simulink model "LV_grid"  (R2021b)
settings: Solver=VariableStepAuto  StartTime=0  StopTime=5.0005  FixedStep=5e-4  RelTol=1e-3
model workspace (MAT data in the model file):
  P2_1 = 3450
  idx = 1
  time_counter = 1
libraries: spsGroundLib x97, spsStairGeneratorLib x96, spsPiSectionLineLib x90, spsThreePhasePISectionLineLib x90, spsVariableInductorLib x48, spsVariableResistorLib x48, spsRMSLib x36, spsThreePhaseVIMeasurementLib x34, spsACVoltageSourceLib x5, spsLinearTransformerLib x5, spsPower3phInstantaneousLib x1, spsThreePhaseMutualInductanceZ1Z0Lib x1
(part 1 of 6)
settings Model: Creator=vasri  LastModifiedBy=vasri
settings SolverCC: AlgebraicLoopSolver=TrustRegion
settings DataIOCC: FinalStateName=LV_grid_ctx01  SaveFinalState=on  SaveOperatingPoint=on
settings DebuggingCC: SFMachineParentedDataDiag=warning

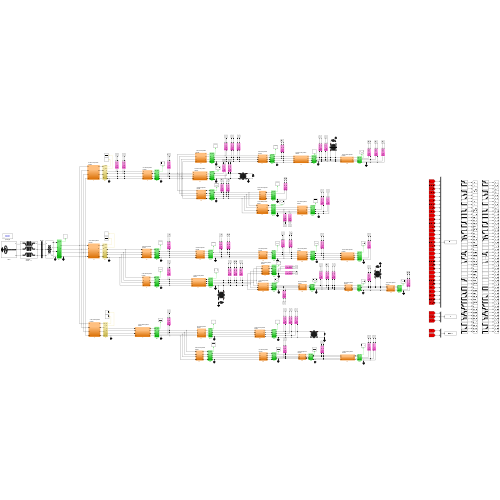
[thumbnail: Simulink's stored preview of the top-level diagram]
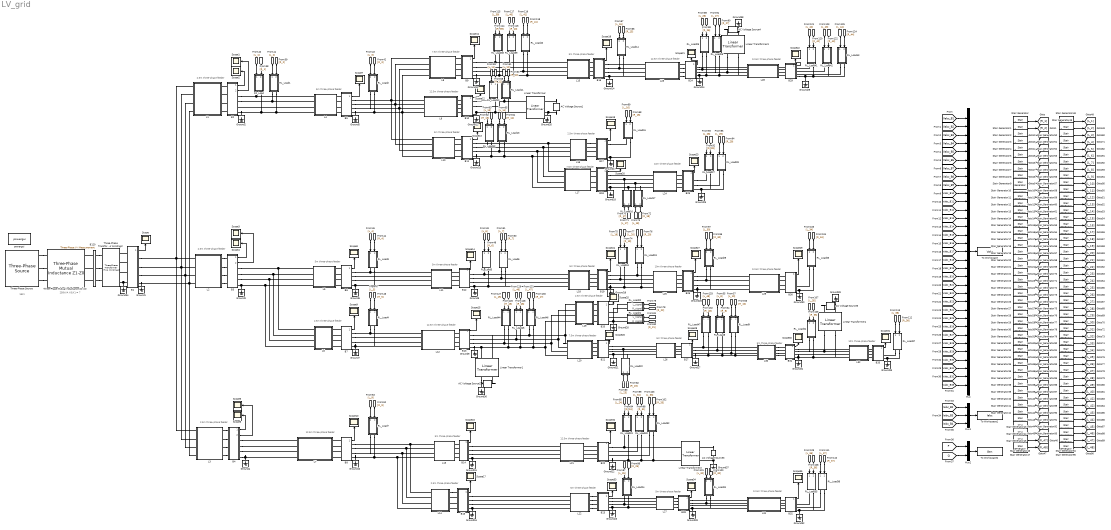
== system LV_grid ==
  note: 12.5m three-phase
      | feeder
  note: 2.5m three-phase
      | feeder
  note: 5m three-phase
      | feeder
  note: 15kV
  note: 250kVA
      | Χ0/Χ1 = 7
  note: 7.5m three-phase
      | feeder
  note: 10m three-phase
      | feeder
  note: 2.5m three-phase
      | feeder
  note: 2.5m three-phase
      | feeder
  note: 2.5m three-phase
      | feeder
  note: 2.5m three-phase
      | feeder
  note: 5m three-phase
      | feeder
  note: 5m three-phase
      | feeder
  note: 5m three-phase
      | feeder
  note: 5m three-phase
      | feeder
  note: 5m three-phase
      | feeder
  note: 5m three-phase
      | feeder
  note: 5m three-phase
      | feeder
  note: 5m three-phase
      | feeder
  note: 5m three-phase
      | feeder
  note: 5m three-phase
      | feeder
  note: 7.5m three-phase
      | feeder
  note: 7.5m three-phase
      | feeder
  note: 10m three-phase
      | feeder
  note: 10m three-phase
      | feeder
  note: 12.5m three-phase
      | feeder
  note: 12.5m three-phase
      | feeder
  note: 12.5m three-phase
      | feeder
  note: 12.5m three-phase
      | feeder
  note: 12.5m three-phase
      | feeder
  note: 12.5m three-phase
      | feeder
  note: 12.5m three-phase
      | feeder
  note: 2.5m three-phase
      | feeder
  note: 2.5m three-phase
      | feeder
  " B120" : spsThreePhaseVIMeasurementLib/Three-Phase V-I Measurement  VoltageMeasurement=no  SetLabelV=off  LabelV=Vabc  Vpu=off  VpuLL=off  CurrentMeasurement=no  SetLabelI=off  LabelI=Iabc  Ipu=on  Pbase=100e6  Vbase=1  OutputType=Complex  PhasorSimulation=off  PSBequivalent=0
  AC Voltage Source1 : spsACVoltageSourceLib/AC Voltage Source  Amplitude=325.27  Phase=-120  Frequency=50  SampleTime=0  Measurements=None  BusType=PV  Pref=6596.9588  Qref=0  Qmin=-inf  Qmax=+inf
  AC Voltage Source2 : spsACVoltageSourceLib/AC Voltage Source  Amplitude=325.27  Phase=0  Frequency=50  SampleTime=0  Measurements=None  BusType=PV  Pref=4239.5175  Qref=0  Qmin=-inf  Qmax=+inf
  AC Voltage Source3 : spsACVoltageSourceLib/AC Voltage Source  Amplitude=325.27  Phase=0  Frequency=50  SampleTime=0  Measurements=None  BusType=PV  Pref=2354.85  Qref=0  Qmin=-inf  Qmax=+inf
  AC Voltage Source4 : spsACVoltageSourceLib/AC Voltage Source  Amplitude=325.27  Phase=120  Frequency=50  SampleTime=0  Measurements=None  BusType=PV  Pref=9631.012  Qref=0  Qmin=-inf  Qmax=+inf
  AC Voltage Source5 : spsACVoltageSourceLib/AC Voltage Source  Amplitude=325.27  Phase=-120  Frequency=50  SampleTime=0  Measurements=None  BusType=PV  Pref=3979.8713  Qref=0  Qmin=-inf  Qmax=+inf
  B1 : Subsystem
  B10 : Subsystem
  B11 : Subsystem
  B12 : Subsystem
  B13 : Subsystem
  B14 : Subsystem
  B15 : Subsystem
  B16 : Subsystem
  B17 : Subsystem
  B18 : Subsystem
  B19 : Subsystem
  B2 : Subsystem
  B20 : Subsystem
  B21 : Subsystem
  B22 : Subsystem
  B23 : Subsystem
  B24 : Subsystem
  B25 : Subsystem
  B26 : Subsystem
  B27 : Subsystem
  B28 : Subsystem
  B29 : Subsystem
  B3 : Subsystem
  B30 : Subsystem
  B31 : Subsystem
  B32 : Subsystem
  B33 : Subsystem
  B4 : Subsystem
  B5 : Subsystem
  B6 : Subsystem
  B7 : Subsystem
  B8 : Subsystem
  B9 : Subsystem
  Ground{1..39} (39 alike) : spsGroundLib/Ground  LConnTagsString=a
  L1 : Subsystem
  L10 : Subsystem
  L11 : Subsystem
  L12 : Subsystem
  L13 : Subsystem
  L14 : Subsystem
  L15 : Subsystem
  L16 : Subsystem
  L17 : Subsystem
  L18 : Subsystem
  L19 : Subsystem
  L2 : Subsystem
  L20 : Subsystem
  L21 : Subsystem
  L22 : Subsystem
  L23 : Subsystem
  L24 : Subsystem
  L25 : Subsystem
  L26 : Subsystem
  L27 : Subsystem
  L28 : Subsystem
  L29 : Subsystem
  L3 : Subsystem
  L30 : Subsystem
  L31 : Subsystem
  L32 : Subsystem
  L4 : Subsystem
  L5 : Subsystem
  L6 : Subsystem
  L7 : Subsystem
  L8 : Subsystem
  L9 : Subsystem
  Linear Transformer{,1..4} (5 alike) : spsLinearTransformerLib/Linear Transformer  UNITS=pu  NominalPower=[ 3680 50 ]  winding1="[ 400  0.002  0.08 ]"  winding2="[ 400  0.002  0.08 ]"  ThreeWindings=off  winding3=[ 315e3 0.002 0.08 ]  RmLm=[ 500 500 ]  Measurements=None  DataType=off
  Mux : Mux  Inputs=33
  Mux1 : Mux  Inputs=3
  Mux2 : Mux  Inputs=2
  RL_Load : Subsystem
  RL_Load1 : Subsystem
  RL_Load10 : Subsystem
  RL_Load11 : Subsystem
  RL_Load12 : Subsystem
  RL_Load13 : Subsystem
  RL_Load14 : Subsystem
  RL_Load15 : Subsystem
  RL_Load16 : Subsystem
  RL_Load17 : Subsystem
  RL_Load18 : Subsystem
  RL_Load19 : Subsystem
  RL_Load2 : Subsystem
  RL_Load20 : Subsystem
  RL_Load21 : Subsystem
  RL_Load22 : Subsystem
  RL_Load23 : Subsystem
  RL_Load24 : Subsystem
  RL_Load25 : Subsystem
  RL_Load26 : Subsystem
  RL_Load27 : Subsystem
  RL_Load28 : Subsystem
  RL_Load29 : Subsystem
  RL_Load3 : Subsystem
  RL_Load30 : Subsystem
  RL_Load31 : Subsystem
  RL_Load32 : Subsystem
  RL_Load33 : Subsystem
  RL_Load34 : Subsystem
  RL_Load35 : Subsystem
  RL_Load36 : Subsystem
  RL_Load37 : Subsystem
  RL_Load38 : Subsystem
  RL_Load39 : Subsystem
  RL_Load4 : Subsystem
  RL_Load40 : Subsystem
  RL_Load41 : Subsystem
  RL_Load42 : Subsystem
  RL_Load43 : Subsystem
  RL_Load44 : Subsystem
  RL_Load45 : Subsystem
  RL_Load46 : Subsystem
  RL_Load47 : Subsystem
  RL_Load5 : Subsystem
  RL_Load6 : Subsystem
  RL_Load7 : Subsystem
  RL_Load8 : Subsystem
  RL_Load9 : Subsystem
  Scope{,1..35} (36 alike) : Scope
  Stair Generator : spsStairGeneratorLib/Stair Generator  t=[0,2.617,3.6925,4.8825]  e=[168.7617,168.5927,168.424,168.2557]  Ts=0.0005
  Stair Generator1 : spsStairGeneratorLib/Stair Generator  t=[0,1.0365,2.15]  e=[73.2041,70.2093,67.4499]  Ts=0.0005
  Stair Generator10 : spsStairGeneratorLib/Stair Generator  t=[0,1.492,2.483]  e=[35.5387,35.625,35.7117]  Ts=0.0005
  Stair Generator11 : spsStairGeneratorLib/Stair Generator  t=[0,2.5075,4.45]  e=[24.3172,26.1566,28.2971]  Ts=0.0005
  Stair Generator12 : spsStairGeneratorLib/Stair Generator  t=[0,1.3855]  e=[0,0]  Ts=0.0005
  Stair Generator13 : spsStairGeneratorLib/Stair Generator  t=[0,0.0745,2.0645,2.6705,2.8715]  e=[353.8462,353.7729,353.6997,353.6265,353.5533]  Ts=0.0005
  Stair Generator14 : spsStairGeneratorLib/Stair Generator  t=[0,2.534,3.5145]  e=[220.7485,220.5687,220.3893]  Ts=0.0005
  Stair Generator15 : spsStairGeneratorLib/Stair Generator  t=[0,0.325,1.7935,1.907]  e=[979.2809,980.7642,982.2521,983.7445]  Ts=0.0005
  Stair Generator16 : spsStairGeneratorLib/Stair Generator  t=[0,1.018,1.172,1.9675,4.0695]  e=[234.6084,234.5768,234.5452,234.5136,234.4821]  Ts=0.0005
  Stair Generator17 : spsStairGeneratorLib/Stair Generator  t=[0,0.2685,1.876,3.8755]  e=[98.0581,98.0807,98.1032,98.1258]  Ts=0.0005
  Stair Generator18 : spsStairGeneratorLib/Stair Generator  t=[0,0.827,1.5965,4.5615]  e=[253.6736,253.7195,253.7655,253.8114]  Ts=0.0005
  Stair Generator19 : spsStairGeneratorLib/Stair Generator  t=[0,1.6495]  e=[0,0]  Ts=0.0005
  Stair Generator2 : spsStairGeneratorLib/Stair Generator  t=[0,1.6175]  e=[0,0]  Ts=0.0005
  Stair Generator20 : spsStairGeneratorLib/Stair Generator  t=[0,0.3505,1.0215,3.8365]  e=[6.1612,6.1612,6.1612,6.1612]  Ts=0.0005
  Stair Generator21 : spsStairGeneratorLib/Stair Generator  t=[0,0.7915,1.4325,3.436,4.7505]  e=[113.7634,113.7634,113.7634,113.7634,113.7634]  Ts=0.0005
  Stair Generator22 : spsStairGeneratorLib/Stair Generator  t=[0,0.706,2.561,3.607]  e=[126.7148,126.7293,126.7438,126.7584]  Ts=0.0005
  Stair Generator23 : spsStairGeneratorLib/Stair Generator  t=[0,2.037,3.661,3.7495,4.6445]  e=[58.0436,58.0068,57.9701,57.9334,57.8968]  Ts=0.0005
  Stair Generator24 : spsStairGeneratorLib/Stair Generator  t=[0,1.096,1.198,2.605,4.2125]  e=[288.4476,288.4443,288.4409,288.4376,288.4343]  Ts=0.0005
  Stair Generator25 : spsStairGeneratorLib/Stair Generator  t=[0,2.346,3.315,3.97,4.0815]  e=[48.1074,48.1096,48.1118,48.114,48.1162]  Ts=0.0005
  Stair Generator26 : spsStairGeneratorLib/Stair Generator  t=[0,1.548]  e=[0,0]  Ts=0.0005
  Stair Generator27 : spsStairGeneratorLib/Stair Generator  t=[0,3.4385]  e=[0,0]  Ts=0.0005
  Stair Generator28 : spsStairGeneratorLib/Stair Generator  t=[0,3.85,4.935]  e=[230,230,230]  Ts=0.0005
  Stair Generator29 : spsStairGeneratorLib/Stair Generator  t=[0,4.1485]  e=[0,0]  Ts=0.0005
  Stair Generator3 : spsStairGeneratorLib/Stair Generator  t=[0,0.555,1.65,1.8765]  e=[79.1582,78.7659,78.3775,77.9928]  Ts=0.0005
  Stair Generator30 : spsStairGeneratorLib/Stair Generator  t=[0,2.977,3.531]  e=[172.8758,172.8758,172.8758]  Ts=0.0005
  Stair Generator31 : spsStairGeneratorLib/Stair Generator  t=[0,0.3405,2.484,3.765,4.326]  e=[231.0087,231.008,231.0073,231.0067,231.006]  Ts=0.0005
  Stair Generator32 : spsStairGeneratorLib/Stair Generator  t=[0,4.843]  e=[0,0]  Ts=0.0005
  Stair Generator33 : spsStairGeneratorLib/Stair Generator  t=[0,0.4945,2.7355]  e=[78.2464,78.4776,78.7101]  Ts=0.0005
  Stair Generator34 : spsStairGeneratorLib/Stair Generator  t=[0,0.5355,2.0155]  e=[152.2068,152.1819,152.157]  Ts=0.0005
  Stair Generator35 : spsStairGeneratorLib/Stair Generator  t=[0,2.8335,3.069,3.6215,3.9155]  e=[145.2339,145.2378,145.2418,145.2458,145.2498]  Ts=0.0005
  Stair Generator36 : spsStairGeneratorLib/Stair Generator  t=[0,2.8845,4.057,4.358,4.7205]  e=[111.5724,111.5869,111.6013,111.6158,111.6302]  Ts=0.0005
  Stair Generator37 : spsStairGeneratorLib/Stair Generator  t=[0,2.5385,3.9445]  e=[80.107,80.0996,80.0922]  Ts=0.0005
  Stair Generator38 : spsStairGeneratorLib/Stair Generator  t=[0,2.3655,4.1445]  e=[131.3855,131.1249,130.8652]  Ts=0.0005
  Stair Generator39 : spsStairGeneratorLib/Stair Generator  t=[0,0.3645,1.3915,1.613,4.881]  e=[129.739,129.4059,129.0744,128.7447,128.4166]  Ts=0.0005
  Stair Generator4 : spsStairGeneratorLib/Stair Generator  t=[0,1.711,2.659,4.086]  e=[59.9269,59.9317,59.9365,59.9413]  Ts=0.0005
  Stair Generator40 : spsStairGeneratorLib/Stair Generator  t=[0,3.7565,4.1565,4.612]  e=[61.3324,61.3175,61.3027,61.2879]  Ts=0.0005
  Stair Generator41 : spsStairGeneratorLib/Stair Generator  t=[0,1.6355,2.692,4.021]  e=[60.1003,60.1377,60.1751,60.2126]  Ts=0.0005
  Stair Generator42 : spsStairGeneratorLib/Stair Generator  t=[0,0.382,2.317,4.1045,4.76]  e=[105.4187,105.3985,105.3784,105.3582,105.3381]  Ts=0.0005
  Stair Generator43 : spsStairGeneratorLib/Stair Generator  t=[0,1.175,1.995,3.544]  e=[54.3782,56.0322,57.7901,59.6618]  Ts=0.0005
  Stair Generator44 : spsStairGeneratorLib/Stair Generator  t=[0,1.341,3.2495,4.163,4.9775]  e=[134.6056,134.6056,134.6056,134.6056,134.6056]  Ts=0.0005
  Stair Generator45 : spsStairGeneratorLib/Stair Generator  t=[0,3.5205,4.662]  e=[38.2589,37.6587,37.077]  Ts=0.0005
  Stair Generator46 : spsStairGeneratorLib/Stair Generator  t=[0,1.9045,2.8425,3.1735,3.439]  e=[221.8029,221.8317,221.8605,221.8893,221.9182]  Ts=0.0005
  Stair Generator47 : spsStairGeneratorLib/Stair Generator  t=[0,1.8165,2.0385]  e=[121.7591,121.7699,121.7806]  Ts=0.0005
  Stair Generator48 : spsStairGeneratorLib/Stair Generator  t=[0,2.617,3.6925,4.8825]  e=[1.6344,1.6327,1.6311,1.6295]  Ts=0.0005
  Stair Generator49 : spsStairGeneratorLib/Stair Generator  t=[0,1.0365,2.15]  e=[0.70894,0.67993,0.65321]  Ts=0.0005
  Stair Generator5 : spsStairGeneratorLib/Stair Generator  t=[0,0.602,2.606,3.128,3.872]  e=[17.5487,17.8286,18.1176,18.4162,18.7247]  Ts=0.0005
  Stair Generator50 : spsStairGeneratorLib/Stair Generator  t=[0,1.6175]  e=[0,0]  Ts=0.0005
  Stair Generator51 : spsStairGeneratorLib/Stair Generator  t=[0,0.555,1.65,1.8765]  e=[0.7666,0.7628,0.75904,0.75531]  Ts=0.0005
  Stair Generator52 : spsStairGeneratorLib/Stair Generator  t=[0,1.711,2.659,4.086]  e=[0.58035,0.5804,0.58045,0.58049]  Ts=0.0005
  Stair Generator53 : spsStairGeneratorLib/Stair Generator  t=[0,0.602,2.606,3.128,3.872]  e=[0.16995,0.17266,0.17546,0.17835,0.18134]  Ts=0.0005
  Stair Generator54 : spsStairGeneratorLib/Stair Generator  t=[0,1.7335]  e=[0,0]  Ts=0.0005
  Stair Generator55 : spsStairGeneratorLib/Stair Generator  t=[0,1.6735,2.8735]  e=[0.73112,0.73068,0.73024]  Ts=0.0005
  Stair Generator56 : spsStairGeneratorLib/Stair Generator  t=[0,4.32]  e=[0,0]  Ts=0.0005
  Stair Generator57 : spsStairGeneratorLib/Stair Generator  t=[0,0.9935,0.9965,3.363,4.5095]  e=[0.43413,0.43425,0.43436,0.43448,0.4346]  Ts=0.0005
  Stair Generator58 : spsStairGeneratorLib/Stair Generator  t=[0,1.492,2.483]  e=[0.34417,0.34501,0.34585]  Ts=0.0005
  Stair Generator59 : spsStairGeneratorLib/Stair Generator  t=[0,2.5075,4.45]  e=[0.2355,0.25331,0.27404]  Ts=0.0005
  Stair Generator6 : spsStairGeneratorLib/Stair Generator  t=[0,1.7335]  e=[0,0]  Ts=0.0005
  Stair Generator60 : spsStairGeneratorLib/Stair Generator  t=[0,1.3855]  e=[0,0]  Ts=0.0005
  Stair Generator61 : spsStairGeneratorLib/Stair Generator  t=[0,0.0745,2.0645,2.6705,2.8715]  e=[3.4268,3.4261,3.4254,3.4246,3.4239]  Ts=0.0005
  Stair Generator62 : spsStairGeneratorLib/Stair Generator  t=[0,2.534,3.5145]  e=[2.1378,2.1361,2.1343]  Ts=0.0005
  Stair Generator63 : spsStairGeneratorLib/Stair Generator  t=[0,0.325,1.7935,1.907]  e=[9.4837,9.4981,9.5125,9.5269]  Ts=0.0005
  Stair Generator64 : spsStairGeneratorLib/Stair Generator  t=[0,1.018,1.172,1.9675,4.0695]  e=[2.272,2.2717,2.2714,2.2711,2.2708]  Ts=0.0005
  Stair Generator65 : spsStairGeneratorLib/Stair Generator  t=[0,0.2685,1.876,3.8755]  e=[0.94963,0.94985,0.95007,0.95029]  Ts=0.0005
  Stair Generator66 : spsStairGeneratorLib/Stair Generator  t=[0,0.827,1.5965,4.5615]  e=[2.4567,2.4571,2.4576,2.458]  Ts=0.0005
  Stair Generator67 : spsStairGeneratorLib/Stair Generator  t=[0,1.6495]  e=[0,0]  Ts=0.0005
  Stair Generator68 : spsStairGeneratorLib/Stair Generator  t=[0,0.3505,1.0215,3.8365]  e=[0.059667,0.059667,0.059667,0.059667]  Ts=0.0005
  Stair Generator69 : spsStairGeneratorLib/Stair Generator  t=[0,0.7915,1.4325,3.436,4.7505]  e=[1.1017,1.1017,1.1017,1.1017,1.1017]  Ts=0.0005
  Stair Generator7 : spsStairGeneratorLib/Stair Generator  t=[0,1.6735,2.8735]  e=[75.4947,75.4495,75.4044]  Ts=0.0005
  Stair Generator70 : spsStairGeneratorLib/Stair Generator  t=[0,0.706,2.561,3.607]  e=[1.2272,1.2273,1.2274,1.2276]  Ts=0.0005
  Stair Generator71 : spsStairGeneratorLib/Stair Generator  t=[0,2.037,3.661,3.7495,4.6445]  e=[0.56212,0.56176,0.5614,0.56105,0.56069]  Ts=0.0005
  Stair Generator72 : spsStairGeneratorLib/Stair Generator  t=[0,1.096,1.198,2.605,4.2125]  e=[2.7934,2.7934,2.7934,2.7933,2.7933]  Ts=0.0005
  Stair Generator73 : spsStairGeneratorLib/Stair Generator  t=[0,2.346,3.315,3.97,4.0815]  e=[0.46589,0.46591,0.46593,0.46595,0.46598]  Ts=0.0005
  Stair Generator74 : spsStairGeneratorLib/Stair Generator  t=[0,1.548]  e=[0,0]  Ts=0.0005
  Stair Generator75 : spsStairGeneratorLib/Stair Generator  t=[0,3.4385]  e=[0,0]  Ts=0.0005
  Stair Generator76 : spsStairGeneratorLib/Stair Generator  t=[0,3.85,4.935]  e=[2.2274,2.2274,2.2274]  Ts=0.0005
  Stair Generator77 : spsStairGeneratorLib/Stair Generator  t=[0,4.1485]  e=[0,0]  Ts=0.0005
  Stair Generator78 : spsStairGeneratorLib/Stair Generator  t=[0,2.977,3.531]  e=[1.6742,1.6742,1.6742]  Ts=0.0005
  Stair Generator79 : spsStairGeneratorLib/Stair Generator  t=[0,0.3405,2.484,3.765,4.326]  e=[2.2372,2.2372,2.2372,2.2372,2.2371]  Ts=0.0005
  Stair Generator8 : spsStairGeneratorLib/Stair Generator  t=[0,4.32]  e=[0,0]  Ts=0.0005
  Stair Generator80 : spsStairGeneratorLib/Stair Generator  t=[0,4.843]  e=[0,0]  Ts=0.0005
  Stair Generator81 : spsStairGeneratorLib/Stair Generator  t=[0,0.4945,2.7355]  e=[0.75777,0.76001,0.76226]  Ts=0.0005
  Stair Generator82 : spsStairGeneratorLib/Stair Generator  t=[0,0.5355,2.0155]  e=[1.474,1.4738,1.4735]  Ts=0.0005
  Stair Generator83 : spsStairGeneratorLib/Stair Generator  t=[0,2.8335,3.069,3.6215,3.9155]  e=[1.4065,1.4065,1.4066,1.4066,1.4067]  Ts=0.0005
  Stair Generator84 : spsStairGeneratorLib/Stair Generator  t=[0,2.8845,4.057,4.358,4.7205]  e=[1.0805,1.0806,1.0808,1.0809,1.0811]  Ts=0.0005
  Stair Generator85 : spsStairGeneratorLib/Stair Generator  t=[0,2.5385,3.9445]  e=[0.77579,0.77571,0.77564]  Ts=0.0005
  Stair Generator86 : spsStairGeneratorLib/Stair Generator  t=[0,2.3655,4.1445]  e=[1.2724,1.2699,1.2673]  Ts=0.0005
  Stair Generator87 : spsStairGeneratorLib/Stair Generator  t=[0,0.3645,1.3915,1.613,4.881]  e=[1.2564,1.2532,1.25,1.2468,1.2436]  Ts=0.0005
  Stair Generator88 : spsStairGeneratorLib/Stair Generator  t=[0,3.7565,4.1565,4.612]  e=[0.59397,0.59382,0.59368,0.59353]  Ts=0.0005
  Stair Generator89 : spsStairGeneratorLib/Stair Generator  t=[0,1.6355,2.692,4.021]  e=[0.58203,0.5824,0.58276,0.58312]  Ts=0.0005
  Stair Generator9 : spsStairGeneratorLib/Stair Generator  t=[0,0.9935,0.9965,3.363,4.5095]  e=[44.8279,44.84,44.8521,44.8642,44.8764]  Ts=0.0005
  Stair Generator90 : spsStairGeneratorLib/Stair Generator  t=[0,0.382,2.317,4.1045,4.76]  e=[1.0209,1.0207,1.0205,1.0203,1.0201]  Ts=0.0005
  Stair Generator91 : spsStairGeneratorLib/Stair Generator  t=[0,1.175,1.995,3.544]  e=[0.52662,0.54264,0.55966,0.57779]  Ts=0.0005
  Stair Generator92 : spsStairGeneratorLib/Stair Generator  t=[0,1.341,3.2495,4.163,4.9775]  e=[1.3036,1.3036,1.3036,1.3036,1.3036]  Ts=0.0005
  Stair Generator93 : spsStairGeneratorLib/Stair Generator  t=[0,3.5205,4.662]  e=[0.37051,0.3647,0.35907]  Ts=0.0005
  Stair Generator94 : spsStairGeneratorLib/Stair Generator  t=[0,1.9045,2.8425,3.1735,3.439]  e=[2.148,2.1483,2.1486,2.1489,2.1491]  Ts=0.0005
  Stair Generator95 : spsStairGeneratorLib/Stair Generator  t=[0,1.8165,2.0385]  e=[1.1792,1.1793,1.1794]  Ts=0.0005
  Three-Phase Mutual Inductance Z1-Z0 : spsThreePhaseMutualInductanceZ1Z0Lib/Three-Phase Mutual Inductance Z1-Z0  LConnTagsString=a|b|c  RConnTagsString=A|B|C  PositiveSequence="[ 2  50e-3]"  ZeroSequence="[ 14  350e-3]"
      settings: AttributesFormatString=\n  SourceProductBaseCode=PS
  Three-Phase Transformer (Two Windings) : spsThreePhaseTransformerTwoWindingsLib/Three-Phase Transformer (Two Windings)  Winding1Connection=Yg  Winding2Connection=Yn  CoreType=Three single-phase transformers  SetSaturation=off  Hysteresis=off  DataFile='hysteresis'  SetInitialFlux=off  Measurements=None  UNITS=pu  NominalPower=[ 250e3 , 50 ]  Winding1=[15e3 0.002 0.08]  Winding2=[400 0.002 0.08]  Rm=500  Lm=500  L0=0.5  Saturation=[0 0;0.084835 28.291;35.348 35.835]  InitialFluxes=[0.8 -0.8 0.69999]  BreakLoop=off  DiscreteSolver=Trapezoidal iterative  DataType=off  TransfoNumber=1
  Three-Phase Source : spsThreePhaseSourceLib/Three-Phase Source  InternalConnection=Yg  VoltagePhases=off  Voltage=15e3  PhaseAngle=0  Voltage_phases=[25e3 25e3 25e3]/sqrt(3)  PhaseAngles_phases=[0 -120 +120]  Frequency=50  NonIdealSource=off  SpecifyImpedance=off  Resistance=0  Inductance=0  ShortCircuitLevel=100e6  BaseVoltage=25e3  XRratio=7  BusType=PV  Pref=50e6  Qref=0  Prefabc=[10e3, 10e3, 10e3]  Qrefabc=[0, 0, 0]  Qmin=-inf  Qmax=inf
  To Workspace : ToWorkspace  VariableName=Vabc  SampleTime=20e-3
  To Workspace1 : ToWorkspace  VariableName=Iabc  SampleTime=20e-3
  To Workspace2 : ToWorkspace  VariableName=Gen  SampleTime=20e-3
  powergui : spspowerguiLib/powergui  Priority=1  SimulationMode=Discrete  SampleTime=5e-4  frequency=60  Iterations=50  frequencyindice=50  Pbase=100e6  ErrMax=1e-4  UnitsV=kV  UnitsW=MW  buscounter=0  FunctionMessages=off  echomessages=off  EnableUseOfTLC=off  CurrentSourceSwitches=off  DisableSnubberDevices=off  DisableRonSwitches=off  DisableVfSwitches=off  DisplayEquations=off  AutomaticDiscreteSolvers=off  SolverType=Tustin/Backward Euler (TBE)  Interpol=off  ExternalGateDelay=off  methode=off  Ts=100  x0status=blocks  SPID=on  SwTol=0  HookPort=off  NonlinearTolerance=1e-4  nMaxIteration=100  ContinueOnMaxIteration=off  RestoreLinks=warning  ResistiveCurrentMeasurement=off  Frange=[0:2:500]  Ylog=off  Xlog=on  ShowGrid=off  save=off  variable=ZData  structure=0  ZoomFFT=off  StartTime=0.0  cycles=1  DisplayStyle=1  fundamental=60  FreqAxis=off  MaxFrequency=1000  frequencyindicesteady=1  RmsSteady=2  display=off
  wires:
  [Iabc_B3] -> Mux1/2
  [Vabc_B27] -> Mux/27
  [Vabc_B26] -> Mux/26
  [Vabc_B24] -> Mux/24
  [Vabc_B22] -> Mux/22
  [Vabc_B31] -> Mux/31
  [Vabc_B33] -> Mux/33
  [Vabc_B11] -> Mux/11
  [Vabc_B21] -> Mux/21
  [Vabc_B23] -> Mux/23
  [Vabc_B18] -> Mux/18
  [Vabc_B13] -> Mux/13
  [Vabc_B10] -> Mux/10
  [Vabc_B16] -> Mux/16
  [Vabc_B5] -> Mux/5
  [Vabc_B6] -> Mux/6
  [Vabc_B4] -> Mux/4
  [Vabc_B7] -> Mux/7
  [Vabc_B17] -> Mux/17
  [Vabc_B9] -> Mux/9
  [Iabc_B4] -> Mux1/3
  [Vabc_B25] -> Mux/25
  [Vabc_B30] -> Mux/30
  [Vabc_B32] -> Mux/32
  [Vabc_B1] -> Mux/1
  [Vabc_B19] -> Mux/19
  [Vabc_B14] -> Mux/14
  [Vabc_B15] -> Mux/15
  [Vabc_B12] -> Mux/12
  [Vabc_B20] -> Mux/20
  [Vabc_B8] -> Mux/8
  [Vabc_B3] -> Mux/3
  [Vabc_B29] -> Mux/29
  [Iabc_B2] -> Mux1/1
  [Vabc_B28] -> Mux/28
  [Vabc_B2] -> Mux/2
  Mux1/1 -> To Workspace1/1
  Mux/1 -> To Workspace/1
  B3/1(V_out) -> Scope4/1
  B3/2(I_out) -> Scope3/1
  B4/1(V_out) -> Scope6/1
  B4/2(I_out) -> Scope5/1
  B5/1(V_out) -> Scope7/1
  B6/1(V_out) -> Scope8/1
  B7/1(V_out) -> Scope9/1
  B8/1(V_out) -> Scope10/1
  B9/1(V_out) -> Scope11/1
  B10/1(V_out) -> Scope12/1
  B11/1(V_out) -> Scope13/1
  B12/1(V_out) -> Scope14/1
  B14/1(V_out) -> Scope16/1
  B15/1(V_out) -> Scope17/1
  B16/1(V_out) -> Scope18/1
  B17/1(V_out) -> Scope19/1
  B18/1(V_out) -> Scope20/1
  B24/1(V_out) -> Scope21/1
  B29/1(V_out) -> Scope22/1
  B25/1(V_out) -> Scope23/1
  B19/1(V_out) -> Scope24/1
  B20/1(V_out) -> Scope25/1
  B21/1(V_out) -> Scope26/1
  B26/1(V_out) -> Scope27/1
  B27/1(V_out) -> Scope28/1
  B30/1(V_out) -> Scope29/1
  B31/1(V_out) -> Scope30/1
  B33/1(V_out) -> Scope31/1
  B22/1(V_out) -> Scope32/1
  B23/1(V_out) -> Scope33/1
  B28/1(V_out) -> Scope34/1
  B32/1(V_out) -> Scope35/1
  B13/1(V_out) -> Scope15/1
  Mux2/1 -> To Workspace2/1
  [P] -> Mux2/1
  [Q] -> Mux2/2
  B1/1(V_out) -> Scope/1
  B2/1(I_out) -> Scope2/1
  B2/2(V_out) -> Scope1/1
  Stair Generator/1 -> [R_1]
  Stair Generator1/1 -> [R_2]
  Stair Generator2/1 -> [R_3]
  Stair Generator3/1 -> [R_4]
  Stair Generator4/1 -> [R_5]
  Stair Generator5/1 -> [R_6]
  Stair Generator6/1 -> [R_7]
  Stair Generator12/1 -> [R_13]
  Stair Generator13/1 -> [R_14]
  Stair Generator14/1 -> [R_15]
  Stair Generator15/1 -> [R_16]
  Stair Generator16/1 -> [R_17]
  Stair Generator17/1 -> [R_18]
  Stair Generator18/1 -> [R_19]
  Stair Generator19/1 -> [R_20]
  Stair Generator20/1 -> [R_21]
  Stair Generator21/1 -> [R_22]
  Stair Generator22/1 -> [R_23]
  Stair Generator23/1 -> [R_24]
  Stair Generator24/1 -> [R_25]
  Stair Generator25/1 -> [R_26]
  Stair Generator26/1 -> [R_27]
  Stair Generator27/1 -> [R_28]
  Stair Generator28/1 -> [R_29]
  Stair Generator29/1 -> [R_30]
  Stair Generator30/1 -> [R_31]
  Stair Generator31/1 -> [R_32]
  Stair Generator32/1 -> [R_33]
  Stair Generator33/1 -> [R_34]
  Stair Generator34/1 -> [R_35]
  Stair Generator35/1 -> [R_36]
  Stair Generator36/1 -> [R_37]
  Stair Generator37/1 -> [R_38]
  Stair Generator38/1 -> [R_39]
  Stair Generator39/1 -> [R_40]
  Stair Generator40/1 -> [R_41]
  Stair Generator41/1 -> [R_42]
  Stair Generator42/1 -> [R_43]
  Stair Generator43/1 -> [R_44]
  Stair Generator44/1 -> [R_45]
  Stair Generator45/1 -> [R_46]
  Stair Generator46/1 -> [R_47]
  Stair Generator47/1 -> [R_48]
  Stair Generator89/1 -> [L_42]
  Stair Generator86/1 -> [L_39]
  Stair Generator69/1 -> [L_22]
  Stair Generator55/1 -> [L_8]
  Stair Generator85/1 -> [L_38]
  Stair Generator48/1 -> [L_1]
  Stair Generator88/1 -> [L_41]
  Stair Generator71/1 -> [L_24]
  Stair Generator57/1 -> [L_10]
  Stair Generator87/1 -> [L_40]
  Stair Generator64/1 -> [L_17]
  Stair Generator58/1 -> [L_11]
  Stair Generator94/1 -> [L_47]
  Stair Generator68/1 -> [L_21]
  Stair Generator76/1 -> [L_29]
  Stair Generator59/1 -> [L_12]
  Stair Generator65/1 -> [L_18]
  Stair Generator63/1 -> [L_16]
  Stair Generator56/1 -> [L_9]
  Stair Generator52/1 -> [L_5]
  Stair Generator84/1 -> [L_37]
  Stair Generator60/1 -> [L_13]
  Stair Generator92/1 -> [L_45]
  Stair Generator49/1 -> [L_2]
  Stair Generator82/1 -> [L_35]
  Stair Generator62/1 -> [L_15]
  Stair Generator73/1 -> [L_26]
  Stair Generator81/1 -> [L_34]
  Stair Generator72/1 -> [L_25]
  Stair Generator95/1 -> [L_48]
  Stair Generator93/1 -> [L_46]
  Stair Generator66/1 -> [L_19]
  Stair Generator51/1 -> [L_4]
  Stair Generator90/1 -> [L_43]
  Stair Generator78/1 -> [L_31]
  Stair Generator80/1 -> [L_33]
  Stair Generator75/1 -> [L_28]
  Stair Generator83/1 -> [L_36]
  Stair Generator74/1 -> [L_27]
  Stair Generator91/1 -> [L_44]
  Stair Generator79/1 -> [L_32]
  Stair Generator67/1 -> [L_20]
  Stair Generator50/1 -> [L_3]
  Stair Generator77/1 -> [L_30]
  Stair Generator70/1 -> [L_23]
  Stair Generator54/1 -> [L_7]
  Stair Generator61/1 -> [L_14]
  Stair Generator53/1 -> [L_6]
  [R_1] -> RL_Load/2(R_signal)
  [R_2] -> RL_Load1/2(R_signal)
  [L_1] -> RL_Load/1(L_signal)
  [L_2] -> RL_Load1/1(L_signal)
  [L_3] -> RL_Load2/1(L_signal)
  [R_3] -> RL_Load2/2(R_signal)
  [L_4] -> RL_Load3/1(L_signal)
  [R_4] -> RL_Load3/2(R_signal)
  [R_5] -> RL_Load4/2(R_signal)
  [L_5] -> RL_Load4/1(L_signal)
  [L_6] -> RL_Load5/1(L_signal)
  [R_6] -> RL_Load5/2(R_signal)
  [L_7] -> RL_Load6/1(L_signal)
  [R_7] -> RL_Load6/2(R_signal)
  [R_9] -> RL_Load7/2(R_signal)
  [L_9] -> RL_Load7/1(L_signal)
  [R_8] -> RL_Load8/2(R_signal)
  [L_8] -> RL_Load8/1(L_signal)
  [R_10] -> RL_Load9/2(R_signal)
  [L_10] -> RL_Load9/1(L_signal)
  [R_11] -> RL_Load10/2(R_signal)
  [L_11] -> RL_Load10/1(L_signal)
  [R_12] -> RL_Load11/2(R_signal)
  [L_12] -> RL_Load11/1(L_signal)
  [L_13] -> RL_Load12/1(L_signal)
  [L_14] -> RL_Load13/1(L_signal)
  [R_14] -> RL_Load13/2(R_signal)
  [R_13] -> RL_Load12/2(R_signal)
  [L_15] -> RL_Load14/1(L_signal)
  [R_15] -> RL_Load14/2(R_signal)
  [R_16] -> RL_Load15/2(R_signal)
  [L_16] -> RL_Load15/1(L_signal)
  [R_17] -> RL_Load16/2(R_signal)
  [L_17] -> RL_Load16/1(L_signal)
  [L_18] -> RL_Load17/1(L_signal)
  [R_18] -> RL_Load17/2(R_signal)
  [R_20] -> RL_Load19/2(R_signal)
  [L_20] -> RL_Load19/1(L_signal)
  [L_19] -> RL_Load18/1(L_signal)
  [R_19] -> RL_Load18/2(R_signal)
  [R_21] -> RL_Load21/2(R_signal)
  [L_21] -> RL_Load21/1(L_signal)
  [L_22] -> RL_Load20/1(L_signal)
  [R_22] -> RL_Load20/2(R_signal)
  [L_23] -> RL_Load22/1(L_signal)
  [R_23] -> RL_Load22/2(R_signal)
  [R_24] -> RL_Load23/2(R_signal)
  [L_24] -> RL_Load23/1(L_signal)
  [R_25] -> RL_Load24/2(R_signal)
  [L_25] -> RL_Load24/1(L_signal)
  [R_26] -> RL_Load25/2(R_signal)
  [L_26] -> RL_Load25/1(L_signal)
  [L_27] -> RL_Load26/1(L_signal)
  [R_27] -> RL_Load26/2(R_signal)
  [R_28] -> RL_Load27/2(R_signal)
  [R_29] -> RL_Load28/2(R_signal)
  [L_28] -> RL_Load27/1(L_signal)
  [L_29] -> RL_Load28/1(L_signal)
  [L_30] -> RL_Load29/1(L_signal)
  [R_30] -> RL_Load29/2(R_signal)
  [L_31] -> RL_Load30/1(L_signal)
  [R_31] -> RL_Load30/2(R_signal)
  [L_32] -> RL_Load31/1(L_signal)
  [R_32] -> RL_Load31/2(R_signal)
  [R_33] -> RL_Load32/2(R_signal)
  [L_33] -> RL_Load32/1(L_signal)
  [L_34] -> RL_Load33/1(L_signal)
  [R_34] -> RL_Load33/2(R_signal)
  [L_35] -> RL_Load34/1(L_signal)
  [R_35] -> RL_Load34/2(R_signal)
  [L_36] -> RL_Load35/1(L_signal)
  [R_36] -> RL_Load35/2(R_signal)
  [L_37] -> RL_Load36/1(L_signal)
  [R_37] -> RL_Load36/2(R_signal)
  [L_38] -> RL_Load37/1(L_signal)
  [R_38] -> RL_Load37/2(R_signal)
  [L_39] -> RL_Load38/1(L_signal)
  [R_39] -> RL_Load38/2(R_signal)
  [R_40] -> RL_Load39/2(R_signal)
  [L_40] -> RL_Load39/1(L_signal)
  [R_41] -> RL_Load40/2(R_signal)
  [L_41] -> RL_Load40/1(L_signal)
  [L_42] -> RL_Load41/1(L_signal)
  [R_42] -> RL_Load41/2(R_signal)
  [L_43] -> RL_Load42/1(L_signal)
  [R_43] -> RL_Load42/2(R_signal)
  [L_44] -> RL_Load43/1(L_signal)
  [R_44] -> RL_Load43/2(R_signal)
  [L_45] -> RL_Load44/1(L_signal)
  [R_45] -> RL_Load44/2(R_signal)
  [L_46] -> RL_Load45/1(L_signal)
  [R_46] -> RL_Load45/2(R_signal)
  [L_47] -> RL_Load46/1(L_signal)
  [R_47] -> RL_Load46/2(R_signal)
  [L_48] -> RL_Load47/1(L_signal)
  [R_48] -> RL_Load47/2(R_signal)
  Stair Generator7/1 -> [R_8]
  Stair Generator8/1 -> [R_9]
  Stair Generator9/1 -> [R_10]
  Stair Generator10/1 -> [R_11]
  Stair Generator11/1 -> [R_12]
  connections:
  B12/RConn1 -- RL_Load5/RConn1 -- L18/LConn1
  B12/RConn2 -- RL_Load6/RConn1 -- L18/LConn2
  B7/RConn4 -- RL_Load4/RConn2 -- L12/LConn4 -- Ground7/LConn1
  Ground18/LConn1 -- RL_Load17/RConn2 -- L24/LConn4 -- RL_Load16/RConn2 -- B18/RConn4
  Ground24/LConn1 -- L28/LConn4 -- Linear Transformer3/RConn2 -- RL_Load26/RConn2 -- RL_Load25/RConn2 -- B24/RConn4
  L17/LConn4 -- RL_Load13/RConn2 -- RL_Load12/RConn2 -- B11/RConn4 -- Ground13/LConn1 -- L16/LConn4
  B11/RConn3 -- RL_Load13/RConn1 -- L17/LConn3 -- L16/LConn3
  B9/RConn2 -- RL_Load39/RConn1 -- L15/LConn2
  B30/RConn4 -- RL_Load33/RConn2 -- Ground30/LConn1
  Ground36/LConn1 -- AC Voltage Source2/LConn1 -- Linear Transformer1/LConn2
  B9/RConn4 -- Ground11/LConn1 -- RL_Load38/RConn2 -- RL_Load39/RConn2 -- RL_Load40/RConn2 -- L15/LConn4
  Linear Transformer4/LConn2 -- Ground39/LConn1 -- AC Voltage Source5/LConn1
  B22/RConn1 -- RL_Load23/RConn1 -- Linear Transformer2/RConn1
  B18/RConn3 -- RL_Load17/RConn1 -- L24/LConn3
  B13/RConn3 -- RL_Load44/RConn1 -- L19/LConn3 -- L20/LConn3
  Linear Transformer1/RConn1 -- B13/RConn1 -- RL_Load46/RConn1 -- L19/LConn1 -- L20/LConn1
  B32/RConn4 -- RL_Load36/RConn2 -- RL_Load35/RConn2 -- Ground32/LConn1
  L25/LConn4 -- RL_Load19/RConn2 -- RL_Load18/RConn2 -- Ground19/LConn1 -- B19/RConn4
  L30/LConn1 -- RL_Load47/RConn1 -- B27/RConn1
  B18/RConn2 -- RL_Load16/RConn1 -- L24/LConn2
  Ground8/LConn1 -- RL_Load6/RConn2 -- L18/LConn4 -- RL_Load5/RConn2 -- B12/RConn4
  B21/RConn4 -- RL_Load22/RConn2 -- L26/LConn4 -- Ground21/LConn1
  B21/RConn2 -- RL_Load22/RConn1 -- L26/LConn2
  L16/LConn2 -- B11/RConn2 -- L17/LConn2
  Ground28/LConn1 -- RL_Load31/RConn2 -- L31/LConn4 -- B28/RConn4
  B2/RConn1 -- RL_Load/RConn1 -- L4/LConn1
  Ground15/LConn1 -- L21/LConn4 -- B14/RConn4
  Ground14/LConn1 -- RL_Load14/RConn2 -- L23/LConn4 -- B16/RConn4
  B31/RConn4 -- RL_Load34/RConn2 -- Linear Transformer4/RConn2 -- L32/LConn4 -- Ground31/LConn1
  Ground3/LConn1 -- L5/LConn4 -- L6/LConn4 -- B3/RConn4
  L30/LConn4 -- RL_Load9/RConn2 -- RL_Load47/RConn2 -- Ground27/LConn1 -- B27/RConn4 -- RL_Load8/RConn2
  B24/RConn2 -- RL_Load25/RConn1 -- L28/LConn2
  B33/RConn4 -- RL_Load37/RConn2 -- Ground33/LConn1
  L27/LConn4 -- RL_Load24/RConn2 -- B23/RConn4 -- Ground23/LConn1
  B28/RConn2 -- RL_Load31/RConn1 -- L31/LConn2
  B8/RConn4 -- Ground10/LConn1 -- RL_Load7/RConn2 -- L13/LConn4 -- L14/LConn4
  L10/LConn4 -- RL_Load2/RConn2 -- B5/RConn4 -- Ground5/LConn1 -- L9/LConn4 -- L8/LConn4
  L13/LConn3 -- RL_Load7/RConn1 -- B8/RConn3 -- L14/LConn3
  B27/RConn2 -- RL_Load8/RConn1 -- L30/LConn2
  L17/LConn1 -- RL_Load12/RConn1 -- B11/RConn1 -- L16/LConn1
  B19/RConn2 -- RL_Load18/RConn1 -- L25/LConn2
  L8/LConn1 -- L9/LConn1 -- B5/RConn1 -- L10/LConn1
  L6/LConn2 -- B3/RConn2 -- L5/LConn2
  B27/RConn3 -- RL_Load9/RConn1 -- L30/LConn3
  L6/LConn1 -- B3/RConn1 -- L5/LConn1
  B26/RConn2 -- RL_Load29/RConn1 -- L29/LConn2
  Ground4/LConn1 -- B4/RConn4 -- L7/LConn4
  B1/RConn3 -- L1/LConn3 -- L3/LConn3 -- L2/LConn3
  B20/RConn4 -- RL_Load20/RConn2 -- Ground20/LConn1 -- RL_Load21/RConn2
  B6/RConn1 -- RL_Load3/RConn1 -- L11/LConn1
  B29/RConn4 -- RL_Load43/RConn2 -- RL_Load42/RConn2 -- RL_Load41/RConn2 -- Ground29/LConn1
  B13/RConn2 -- RL_Load45/RConn1 -- L19/LConn2 -- L20/LConn2
  B2/RConn2 -- RL_Load1/RConn1 -- L4/LConn2
  L8/LConn3 -- RL_Load2/RConn1 -- B5/RConn3 -- L9/LConn3 -- L10/LConn3
  L14/LConn1 -- L13/LConn1 -- B8/RConn1
  Ground22/LConn1 -- B22/RConn4 -- RL_Load23/RConn2 -- RL_Load30/RConn2 -- RL_Load32/RConn2 -- Linear Transformer2/RConn2
  Ground25/LConn1 -- RL_Load27/RConn2 -- RL_Load28/RConn2 -- B25/RConn4
  L8/LConn2 -- L9/LConn2 -- B5/RConn2 -- L10/LConn2
  B16/RConn2 -- RL_Load14/RConn1 -- L23/LConn2
  B17/RConn4 -- Ground17/LConn1 -- RL_Load15/RConn2
  B23/RConn3 -- RL_Load24/RConn1 -- L27/LConn3
  Ground16/LConn1 -- L22/LConn4 -- B15/RConn4
  AC Voltage Source3/LConn1 -- Linear Transformer2/LConn2 -- Ground37/LConn1
  Ground6/LConn1 -- RL_Load3/RConn2 -- L11/LConn4 -- B6/RConn4
  Ground12/LConn1 -- RL_Load11/RConn2 -- Linear Transformer/RConn2 -- RL_Load10/RConn2 -- B10/RConn4
  L1/LConn4 -- Ground1/LConn1 -- B1/RConn4 -- L2/LConn4 -- L3/LConn4
  AC Voltage Source1/LConn1 -- Linear Transformer/LConn2 -- Ground35/LConn1
  L20/LConn4 -- RL_Load46/RConn2 -- RL_Load45/RConn2 -- RL_Load44/RConn2 -- Ground9/LConn1 -- B13/RConn4 -- Linear Transformer1/RConn2 -- L19/LConn4
  B7/RConn1 -- RL_Load4/RConn1 -- L12/LConn1
  Ground26/LConn1 -- RL_Load29/RConn2 -- L29/LConn4 -- B26/RConn4
  B9/RConn1 -- RL_Load38/RConn1 -- L15/LConn1
  L6/LConn3 -- L5/LConn3 -- B3/RConn3
  B1/RConn2 -- L1/LConn2 -- L3/LConn2 -- L2/LConn2
  Linear Transformer4/RConn1 -- RL_Load34/RConn1 -- B31/RConn2 -- L32/LConn2
  Ground2/LConn1 -- B2/RConn4 -- RL_Load/RConn2 -- RL_Load1/RConn2 -- L4/LConn4
  B1/RConn1 -- L1/LConn1 -- L3/LConn1 -- L2/LConn1
  B1/LConn1 -- Three-Phase Transformer (Two Windings)/RConn1
  B19/RConn1 -- RL_Load19/RConn1 -- L25/LConn1
  B9/RConn3 -- RL_Load40/RConn1 -- L15/LConn3
  " B120"/RConn1 -- Three-Phase Transformer (Two Windings)/LConn3
  B10/RConn2 -- RL_Load11/RConn1 -- Linear Transformer/RConn1
  L14/LConn2 -- L13/LConn2 -- B8/RConn2
  AC Voltage Source5/RConn1 -- Linear Transformer4/LConn1
  " B120"/LConn2 -- Three-Phase Mutual Inductance Z1-Z0/RConn2
  AC Voltage Source1/RConn1 -- Linear Transformer/LConn1
  AC Voltage Source2/RConn1 -- Linear Transformer1/LConn1
  " B120"/RConn2 -- Three-Phase Transformer (Two Windings)/LConn2
  AC Voltage Source4/RConn1 -- Linear Transformer3/LConn1
  AC Voltage Source3/RConn1 -- Linear Transformer2/LConn1
  Three-Phase Source/RConn3 -- Three-Phase Mutual Inductance Z1-Z0/LConn3
  B1/LConn2 -- Three-Phase Transformer (Two Windings)/RConn2
  Three-Phase Source/RConn2 -- Three-Phase Mutual Inductance Z1-Z0/LConn2
  B4/RConn1 -- L7/LConn1
  B4/RConn2 -- L7/LConn2
  " B120"/RConn3 -- Three-Phase Transformer (Two Windings)/LConn1
  B1/LConn3 -- Three-Phase Transformer (Two Windings)/RConn3
  " B120"/LConn3 -- Three-Phase Mutual Inductance Z1-Z0/RConn1
  Three-Phase Source/RConn1 -- Three-Phase Mutual Inductance Z1-Z0/LConn1
  " B120"/LConn1 -- Three-Phase Mutual Inductance Z1-Z0/RConn3
  B1/LConn4 -- Ground34/LConn1 -- Three-Phase Transformer (Two Windings)/RConn4
  B4/RConn3 -- L7/LConn3
  B2/LConn1 -- L1/RConn1
  B2/LConn2 -- L1/RConn2
  B2/LConn3 -- L1/RConn3
  B2/LConn4 -- L1/RConn4
  L4/LConn3 -- B2/RConn3
  L2/RConn1 -- B3/LConn1
  L2/RConn2 -- B3/LConn2
  L2/RConn3 -- B3/LConn3
  L2/RConn4 -- B3/LConn4
  L3/RConn1 -- B4/LConn1
  L3/RConn3 -- B4/LConn3
  L3/RConn2 -- B4/LConn2
  L3/RConn4 -- B4/LConn4
  B5/LConn1 -- L4/RConn1
  B5/LConn2 -- L4/RConn2
  B5/LConn3 -- L4/RConn3
  B5/LConn4 -- L4/RConn4
  B6/LConn1 -- L5/RConn1
  B6/LConn2 -- L5/RConn2
  B6/LConn3 -- L5/RConn3
  B6/LConn4 -- L5/RConn4
  B6/RConn2 -- L11/LConn2
  B6/RConn3 -- L11/LConn3
  B7/LConn2 -- L6/RConn2
  B7/LConn3 -- L6/RConn3
  B7/LConn4 -- L6/RConn4
  B7/RConn3 -- L12/LConn3
  B7/RConn2 -- L12/LConn2
  B7/LConn1 -- L6/RConn1
  B8/LConn1 -- L7/RConn1
  B8/LConn2 -- L7/RConn2
  B8/LConn3 -- L7/RConn3
  B8/LConn4 -- L7/RConn4
  B9/LConn1 -- L8/RConn1
  B9/LConn2 -- L8/RConn2
  B9/LConn3 -- L8/RConn3
  B9/LConn4 -- L8/RConn4
  B10/LConn1 -- L9/RConn1
  B10/LConn2 -- L9/RConn2
  B10/LConn3 -- L9/RConn3
  B10/LConn4 -- L9/RConn4
  B11/LConn1 -- L10/RConn1
  B11/LConn2 -- L10/RConn2
  B11/LConn3 -- L10/RConn3
  B11/LConn4 -- L10/RConn4
  B12/LConn1 -- L11/RConn1
  B12/LConn2 -- L11/RConn2
  B12/LConn3 -- L11/RConn3
  B12/LConn4 -- L11/RConn4
  B12/RConn3 -- L18/LConn3
  B13/LConn1 -- L12/RConn1
  B13/LConn2 -- L12/RConn2
  B13/LConn3 -- L12/RConn3
  B13/LConn4 -- L12/RConn4
  B14/LConn1 -- L13/RConn1
  B14/LConn2 -- L13/RConn2
  B14/LConn3 -- L13/RConn3
  B14/LConn4 -- L13/RConn4
  B14/RConn1 -- L21/LConn1
  B14/RConn2 -- L21/LConn2
  B14/RConn3 -- L21/LConn3
  B15/LConn2 -- L14/RConn2
  B15/LConn3 -- L14/RConn3
  B15/LConn4 -- L14/RConn4
  L14/RConn1 -- B15/LConn1
  B15/RConn1 -- L22/LConn1
  B15/RConn2 -- L22/LConn2
  B15/RConn3 -- L22/LConn3
  B16/LConn1 -- L15/RConn1
  B16/LConn2 -- L15/RConn2
  B16/LConn3 -- L15/RConn3
  B16/LConn4 -- L15/RConn4
  B16/RConn3 -- L23/LConn3
  B16/RConn1 -- L23/LConn1
  B17/LConn2 -- L16/RConn2
  B17/LConn3 -- L16/RConn3
  B17/LConn4 -- L16/RConn4
  L16/RConn1 -- B17/LConn1
  B18/RConn1 -- L24/LConn1
  B18/LConn4 -- L17/RConn4
  B18/LConn3 -- L17/RConn3
  B18/LConn2 -- L17/RConn2
  B18/LConn1 -- L17/RConn1
  B24/LConn1 -- L23/RConn1
  B24/RConn1 -- L28/LConn1
  B29/LConn1 -- L28/RConn1
  B29/LConn2 -- L28/RConn2
  B29/LConn3 -- L28/RConn3
  B29/LConn4 -- L28/RConn4
  B25/LConn1 -- L24/RConn1
  B25/LConn2 -- L24/RConn2
  B25/LConn3 -- L24/RConn3
  B25/LConn4 -- L24/RConn4
  B19/LConn1 -- L18/RConn1
  B19/LConn2 -- L18/RConn2
  B19/LConn3 -- L18/RConn3
  B19/LConn4 -- L18/RConn4
  B19/RConn3 -- L25/LConn3
  B20/LConn1 -- L19/RConn1
  B20/LConn2 -- L19/RConn2
  B20/LConn3 -- L19/RConn3
  B20/LConn4 -- L19/RConn4
  B21/LConn1 -- L20/RConn1
  B21/LConn2 -- L20/RConn2
  B21/LConn3 -- L20/RConn3
  B21/LConn4 -- L20/RConn4
  B21/RConn3 -- L26/LConn3
  B21/RConn1 -- L26/LConn1
  B26/LConn1 -- L25/RConn1
  B26/LConn2 -- L25/RConn2
  B26/LConn3 -- L25/RConn3
  B26/LConn4 -- L25/RConn4
  B26/RConn1 -- L29/LConn1
  B26/RConn3 -- L29/LConn3
  B27/LConn1 -- L26/RConn1
  B27/LConn2 -- L26/RConn2
  B27/LConn3 -- L26/RConn3
  B27/LConn4 -- L26/RConn4
  B30/LConn1 -- L29/RConn1
  B30/LConn2 -- L29/RConn2
  B30/LConn3 -- L29/RConn3
  B30/LConn4 -- L29/RConn4
  L30/RConn1 -- B31/LConn1
  L30/RConn2 -- B31/LConn2
  L30/RConn3 -- B31/LConn3
  L30/RConn4 -- B31/LConn4
  B31/RConn1 -- L32/LConn1
  B31/RConn3 -- L32/LConn3
  B33/LConn1 -- L32/RConn1
  B33/LConn2 -- L32/RConn2
  B33/LConn3 -- L32/RConn3
  B33/LConn4 -- L32/RConn4
  B22/LConn1 -- L21/RConn1
  B22/LConn2 -- L21/RConn2
  B22/LConn3 -- L21/RConn3
  B22/LConn4 -- L21/RConn4
  L22/RConn1 -- B23/LConn1
  L22/RConn2 -- B23/LConn2
  L22/RConn3 -- B23/LConn3
  L22/RConn4 -- B23/LConn4
  B23/RConn1 -- L27/LConn1
  B23/RConn2 -- L27/LConn2
  B28/RConn1 -- L31/LConn1
  B28/RConn3 -- L31/LConn3
  B32/LConn1 -- L31/RConn1
  B32/LConn2 -- L31/RConn2
  B32/LConn3 -- L31/RConn3
  B32/LConn4 -- L31/RConn4
  L23/RConn2 -- B24/LConn2
  L23/RConn3 -- B24/LConn3
  L23/RConn4 -- B24/LConn4
  L28/LConn3 -- RL_Load26/RConn1 -- B24/RConn3 -- Linear Transformer3/RConn1
  L27/RConn4 -- B28/LConn4
  L27/RConn3 -- B28/LConn3
  L27/RConn2 -- B28/LConn2
  L27/RConn1 -- B28/LConn1
  Ground38/LConn1 -- AC Voltage Source4/LConn1 -- Linear Transformer3/LConn2
  B10/RConn1 -- RL_Load10/RConn1
  B17/RConn1 -- RL_Load15/RConn1
  RL_Load21/RConn1 -- B20/RConn3
  RL_Load20/RConn1 -- B20/RConn2
  B25/RConn2 -- RL_Load27/RConn1
  B25/RConn3 -- RL_Load28/RConn1
  RL_Load30/RConn1 -- B22/RConn2
  RL_Load32/RConn1 -- B22/RConn3
  RL_Load33/RConn1 -- B30/RConn3
  RL_Load35/RConn1 -- B32/RConn2
  RL_Load36/RConn1 -- B32/RConn3
  RL_Load37/RConn1 -- B33/RConn3
  RL_Load41/RConn1 -- B29/RConn1
  RL_Load42/RConn1 -- B29/RConn2
  RL_Load43/RConn1 -- B29/RConn3

== system LV_grid/B1 ==
  MATLAB Function : MATLAB Function  TreatAsAtomicUnit=on
  "Power (3ph, Instantaneous)" : spsPower3phInstantaneousLib/Power (3ph, Instantaneous)
  RMS : spsRMSLib/RMS  TrueRMS=on  Freq=50  RMSInit=1  Ts=5e-4
  Three-Phase V-I Measurement : spsThreePhaseVIMeasurementLib/Three-Phase V-I Measurement  VoltageMeasurement=phase-to-ground  SetLabelV=off  LabelV=Vabc_B1  Vpu=on  VpuLL=off  CurrentMeasurement=yes  SetLabelI=off  LabelI=Iabc  Ipu=on  Pbase=250e3  Vbase=400/sqrt(2)  OutputType=Complex  PhasorSimulation=off  PSBequivalent=0
  A : PMIOPort  Side=Left
  B : PMIOPort  Port=2  Side=Left
  C : PMIOPort  Port=3  Side=Left
  "N " : PMIOPort  Tag=PMCPort  Port=4  Side=Left
  a : PMIOPort  Tag=PMCPort  Port=5  Side=Right
  b : PMIOPort  Tag=PMCPort  Port=6  Side=Right
  c : PMIOPort  Tag=PMCPort  Port=7  Side=Right
  n : PMIOPort  Tag=PMCPort  Port=8  Side=Right
  V_out : Outport
  tag scope: P=global, Q=global, Vabc_B1=global
  wires:
  Three-Phase V-I Measurement/1 -> RMS/1, "Power (3ph, Instantaneous)"/1
  Three-Phase V-I Measurement/2 -> "Power (3ph, Instantaneous)"/2
  "Power (3ph, Instantaneous)"/1 -> [P]
  "Power (3ph, Instantaneous)"/2 -> [Q]
  RMS/1 -> MATLAB Function/1(u)
  MATLAB Function/1(y) -> V_out/1, [Vabc_B1]
  connections:
  A/RConn1 -- Three-Phase V-I Measurement/LConn1
  B/RConn1 -- Three-Phase V-I Measurement/LConn2
  C/RConn1 -- Three-Phase V-I Measurement/LConn3
  a/RConn1 -- Three-Phase V-I Measurement/RConn1
  b/RConn1 -- Three-Phase V-I Measurement/RConn2
  c/RConn1 -- Three-Phase V-I Measurement/RConn3
  n/RConn1 -- "N "/RConn1

== system LV_grid/B10 ==
  MATLAB Function : MATLAB Function  TreatAsAtomicUnit=on
  RMS : spsRMSLib/RMS  TrueRMS=on  Freq=50  RMSInit=1  Ts=5e-4
  Three-Phase V-I Measurement : spsThreePhaseVIMeasurementLib/Three-Phase V-I Measurement  VoltageMeasurement=phase-to-ground  SetLabelV=off  LabelV=Vabc_B1  Vpu=on  VpuLL=off  CurrentMeasurement=no  SetLabelI=off  LabelI=Iabc  Ipu=off  Pbase=100e6  Vbase=400/sqrt(2)  OutputType=Complex  PhasorSimulation=off  PSBequivalent=0
  A : PMIOPort  Side=Left
  B : PMIOPort  Port=2  Side=Left
  C : PMIOPort  Port=3  Side=Left
  "N " : PMIOPort  Tag=PMCPort  Port=4  Side=Left
  a : PMIOPort  Tag=PMCPort  Port=5  Side=Right
  b : PMIOPort  Tag=PMCPort  Port=6  Side=Right
  c : PMIOPort  Tag=PMCPort  Port=7  Side=Right
  n : PMIOPort  Tag=PMCPort  Port=8  Side=Right
  V_out : Outport
  tag scope: Vabc_B10=global
  wires:
  Three-Phase V-I Measurement/1 -> RMS/1
  RMS/1 -> MATLAB Function/1(u)
  MATLAB Function/1(y) -> [Vabc_B10], V_out/1
  connections:
  A/RConn1 -- Three-Phase V-I Measurement/LConn1
  B/RConn1 -- Three-Phase V-I Measurement/LConn2
  C/RConn1 -- Three-Phase V-I Measurement/LConn3
  a/RConn1 -- Three-Phase V-I Measurement/RConn1
  b/RConn1 -- Three-Phase V-I Measurement/RConn2
  c/RConn1 -- Three-Phase V-I Measurement/RConn3
  n/RConn1 -- "N "/RConn1

== system LV_grid/B11 ==
  MATLAB Function : MATLAB Function  TreatAsAtomicUnit=on
  RMS : spsRMSLib/RMS  TrueRMS=on  Freq=50  RMSInit=1  Ts=5e-4
  Three-Phase V-I Measurement : spsThreePhaseVIMeasurementLib/Three-Phase V-I Measurement  VoltageMeasurement=phase-to-ground  SetLabelV=off  LabelV=Vabc_B1  Vpu=on  VpuLL=off  CurrentMeasurement=no  SetLabelI=off  LabelI=Iabc  Ipu=off  Pbase=100e6  Vbase=400/sqrt(2)  OutputType=Complex  PhasorSimulation=off  PSBequivalent=0
  A : PMIOPort  Side=Left
  B : PMIOPort  Port=2  Side=Left
  C : PMIOPort  Port=3  Side=Left
  "N " : PMIOPort  Tag=PMCPort  Port=4  Side=Left
  a : PMIOPort  Tag=PMCPort  Port=5  Side=Right
  b : PMIOPort  Tag=PMCPort  Port=6  Side=Right
  c : PMIOPort  Tag=PMCPort  Port=7  Side=Right
  n : PMIOPort  Tag=PMCPort  Port=8  Side=Right
  V_out : Outport
  tag scope: Vabc_B11=global
  wires:
  Three-Phase V-I Measurement/1 -> RMS/1
  RMS/1 -> MATLAB Function/1(u)
  MATLAB Function/1(y) -> [Vabc_B11], V_out/1
  connections:
  A/RConn1 -- Three-Phase V-I Measurement/LConn1
  B/RConn1 -- Three-Phase V-I Measurement/LConn2
  C/RConn1 -- Three-Phase V-I Measurement/LConn3
  a/RConn1 -- Three-Phase V-I Measurement/RConn1
  b/RConn1 -- Three-Phase V-I Measurement/RConn2
  c/RConn1 -- Three-Phase V-I Measurement/RConn3
  n/RConn1 -- "N "/RConn1

== system LV_grid/B12 ==
  MATLAB Function : MATLAB Function  TreatAsAtomicUnit=on
  RMS : spsRMSLib/RMS  TrueRMS=on  Freq=50  RMSInit=1  Ts=5e-4
  Three-Phase V-I Measurement : spsThreePhaseVIMeasurementLib/Three-Phase V-I Measurement  VoltageMeasurement=phase-to-ground  SetLabelV=off  LabelV=Vabc_B1  Vpu=on  VpuLL=off  CurrentMeasurement=no  SetLabelI=off  LabelI=Iabc  Ipu=off  Pbase=100e6  Vbase=400/sqrt(2)  OutputType=Complex  PhasorSimulation=off  PSBequivalent=0
  A : PMIOPort  Side=Left
  B : PMIOPort  Port=2  Side=Left
  C : PMIOPort  Port=3  Side=Left
  "N " : PMIOPort  Tag=PMCPort  Port=4  Side=Left
  a : PMIOPort  Tag=PMCPort  Port=5  Side=Right
  b : PMIOPort  Tag=PMCPort  Port=6  Side=Right
  c : PMIOPort  Tag=PMCPort  Port=7  Side=Right
  n : PMIOPort  Tag=PMCPort  Port=8  Side=Right
  V_out : Outport
  tag scope: Vabc_B12=global
  wires:
  Three-Phase V-I Measurement/1 -> RMS/1
  RMS/1 -> MATLAB Function/1(u)
  MATLAB Function/1(y) -> [Vabc_B12], V_out/1
  connections:
  A/RConn1 -- Three-Phase V-I Measurement/LConn1
  B/RConn1 -- Three-Phase V-I Measurement/LConn2
  C/RConn1 -- Three-Phase V-I Measurement/LConn3
  a/RConn1 -- Three-Phase V-I Measurement/RConn1
  b/RConn1 -- Three-Phase V-I Measurement/RConn2
  c/RConn1 -- Three-Phase V-I Measurement/RConn3
  n/RConn1 -- "N "/RConn1

== system LV_grid/B13 ==
  MATLAB Function : MATLAB Function  TreatAsAtomicUnit=on
  RMS : spsRMSLib/RMS  TrueRMS=on  Freq=50  RMSInit=1  Ts=5e-4
  Three-Phase V-I Measurement : spsThreePhaseVIMeasurementLib/Three-Phase V-I Measurement  VoltageMeasurement=phase-to-ground  SetLabelV=off  LabelV=Vabc_B1  Vpu=on  VpuLL=off  CurrentMeasurement=no  SetLabelI=off  LabelI=Iabc  Ipu=off  Pbase=100e6  Vbase=400/sqrt(2)  OutputType=Complex  PhasorSimulation=off  PSBequivalent=0
  A : PMIOPort  Side=Left
  B : PMIOPort  Port=2  Side=Left
  C : PMIOPort  Port=3  Side=Left
  "N " : PMIOPort  Tag=PMCPort  Port=4  Side=Left
  a : PMIOPort  Tag=PMCPort  Port=5  Side=Right
  b : PMIOPort  Tag=PMCPort  Port=6  Side=Right
  c : PMIOPort  Tag=PMCPort  Port=7  Side=Right
  n : PMIOPort  Tag=PMCPort  Port=8  Side=Right
  V_out : Outport
  tag scope: Vabc_B13=global
  wires:
  Three-Phase V-I Measurement/1 -> RMS/1
  RMS/1 -> MATLAB Function/1(u)
  MATLAB Function/1(y) -> [Vabc_B13], V_out/1
  connections:
  A/RConn1 -- Three-Phase V-I Measurement/LConn1
  B/RConn1 -- Three-Phase V-I Measurement/LConn2
  C/RConn1 -- Three-Phase V-I Measurement/LConn3
  a/RConn1 -- Three-Phase V-I Measurement/RConn1
  b/RConn1 -- Three-Phase V-I Measurement/RConn2
  c/RConn1 -- Three-Phase V-I Measurement/RConn3
  n/RConn1 -- "N "/RConn1

== system LV_grid/B14 ==
  MATLAB Function : MATLAB Function  TreatAsAtomicUnit=on
  RMS : spsRMSLib/RMS  TrueRMS=on  Freq=50  RMSInit=1  Ts=5e-4
  Three-Phase V-I Measurement : spsThreePhaseVIMeasurementLib/Three-Phase V-I Measurement  VoltageMeasurement=phase-to-ground  SetLabelV=off  LabelV=Vabc_B1  Vpu=on  VpuLL=off  CurrentMeasurement=no  SetLabelI=off  LabelI=Iabc  Ipu=off  Pbase=100e6  Vbase=400/sqrt(2)  OutputType=Complex  PhasorSimulation=off  PSBequivalent=0
  A : PMIOPort  Side=Left
  B : PMIOPort  Port=2  Side=Left
  C : PMIOPort  Port=3  Side=Left
  "N " : PMIOPort  Tag=PMCPort  Port=4  Side=Left
  a : PMIOPort  Tag=PMCPort  Port=5  Side=Right
  b : PMIOPort  Tag=PMCPort  Port=6  Side=Right
  c : PMIOPort  Tag=PMCPort  Port=7  Side=Right
  n : PMIOPort  Tag=PMCPort  Port=8  Side=Right
  V_out : Outport
  tag scope: Vabc_B14=global
  wires:
  Three-Phase V-I Measurement/1 -> RMS/1
  RMS/1 -> MATLAB Function/1(u)
  MATLAB Function/1(y) -> [Vabc_B14], V_out/1
  connections:
  A/RConn1 -- Three-Phase V-I Measurement/LConn1
  B/RConn1 -- Three-Phase V-I Measurement/LConn2
  C/RConn1 -- Three-Phase V-I Measurement/LConn3
  a/RConn1 -- Three-Phase V-I Measurement/RConn1
  b/RConn1 -- Three-Phase V-I Measurement/RConn2
  c/RConn1 -- Three-Phase V-I Measurement/RConn3
  n/RConn1 -- "N "/RConn1

== system LV_grid/B15 ==
  MATLAB Function : MATLAB Function  TreatAsAtomicUnit=on
  RMS : spsRMSLib/RMS  TrueRMS=on  Freq=50  RMSInit=1  Ts=5e-4
  Three-Phase V-I Measurement : spsThreePhaseVIMeasurementLib/Three-Phase V-I Measurement  VoltageMeasurement=phase-to-ground  SetLabelV=off  LabelV=Vabc_B1  Vpu=on  VpuLL=off  CurrentMeasurement=no  SetLabelI=off  LabelI=Iabc  Ipu=off  Pbase=100e6  Vbase=400/sqrt(2)  OutputType=Complex  PhasorSimulation=off  PSBequivalent=0
  A : PMIOPort  Side=Left
  B : PMIOPort  Port=2  Side=Left
  C : PMIOPort  Port=3  Side=Left
  "N " : PMIOPort  Tag=PMCPort  Port=4  Side=Left
  a : PMIOPort  Tag=PMCPort  Port=5  Side=Right
  b : PMIOPort  Tag=PMCPort  Port=6  Side=Right
  c : PMIOPort  Tag=PMCPort  Port=7  Side=Right
  n : PMIOPort  Tag=PMCPort  Port=8  Side=Right
  V_out : Outport
  tag scope: Vabc_B15=global
  wires:
  Three-Phase V-I Measurement/1 -> RMS/1
  RMS/1 -> MATLAB Function/1(u)
  MATLAB Function/1(y) -> [Vabc_B15], V_out/1
  connections:
  A/RConn1 -- Three-Phase V-I Measurement/LConn1
  B/RConn1 -- Three-Phase V-I Measurement/LConn2
  C/RConn1 -- Three-Phase V-I Measurement/LConn3
  a/RConn1 -- Three-Phase V-I Measurement/RConn1
  b/RConn1 -- Three-Phase V-I Measurement/RConn2
  c/RConn1 -- Three-Phase V-I Measurement/RConn3
  n/RConn1 -- "N "/RConn1
